simulink library "SUB_ECU_L4_MABX_HW_Interface_PIC_PB"  (R2018a)
settings: Solver=VariableStepAuto  StartTime=0.0  StopTime=10.0  RelTol=1e-3
PostLoadFcn:
  | , if any(exist('dsrtsu_mdlpostloadfcn', 'file') == [2, 3, 6]), try dsrtsu_mdlpostloadfcn('Execute', bdroot); catch fprintf('Error in PostLoadFcn (dsrtsu_mdlpostloadfcn) for model "%s":\n %s\n', bdroot, lasterr); end, end,
undefined symbols (not defined in the file or in its folder): CANR_PROPB_REAX_3_13_CHANNEL_APV, CANR_PROPB_REAX_4_13_CHANNEL_APV, CANR_PROPB_XPR_1_50_CHANNEL_APV, ENUM_CAN_RX_T, ENUM_CAN_TX_T, ENUM_REAX_OPERATION_MODE_T, ENUM_SIGNAL_HEALTH_T, ENUM_XBR_CONTROL_MODE_T, ENUM_XBR_EBI_MODE_T, ENUM_XBR_PASS_THROUGH_ACTIVE_T, ENUM_XBR_PRIORITY_T, ENUM_XPR_INHIBIT_PARK_MANUAL_T, ENUM_XPR_INHIBIT_UNPARK_MANUAL_T, ENUM_XPR_PARK_MANUAL_T, ENUM_XPR_UNPARK_MANUAL_T, PROPB_REAX_1_E4_DES_POS_SIG_SRC_APV, PROPB_REAX_1_E4_DESIRED_OPMODE_APV, PROPB_REAX_1_E4_DESIRED_POSITION_APV, PROPB_REAX_CHANNEL_APV, ptc_matlab_lib
libraries: PTC_MBDS_LIB x293, rtican x158, simulink x61, EmE_MBD_Blockset x38, rti1401lib_dio_type4 x14, simulink_need_slupdate x7, $bdroot x5, rti1401lib_adc_type4 x3, rtmapslib x3, dsa_tcpip_lib x2, SUB_ECU_L4_MABX_HW_Interface_PTC_1571 x1, rtitasklib x1
(part 4 of 49)

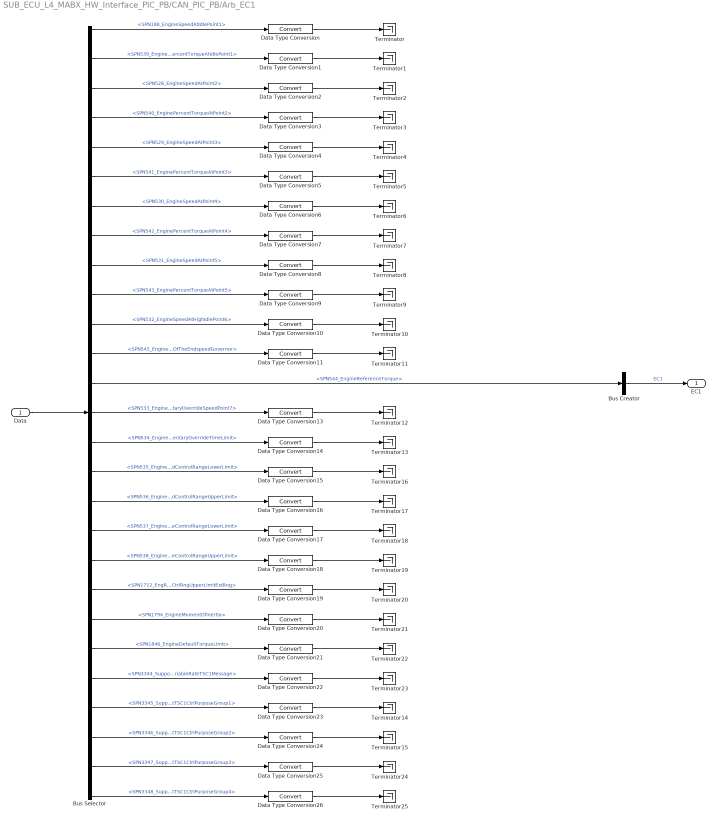
== system SUB_ECU_L4_MABX_HW_Interface_PIC_PB/CAN_PIC_PB/Arb_EC1 ==
  Data : Inport
  Bus Creator : BusCreator  Inputs=1
  Bus Selector : BusSelector  OutputSignals=Signals.SPN188_EngineSpeedAtIdlePoint1,Signals.SPN539_EnginePercentTorqueAtIdlePoint1,Signals.SPN528_EngineSpeedAtPoint2,Signals.SPN540_EnginePercentTorqueAtPoint2,Signals.SPN529_EngineSpeedAtPoint3,Signals.SPN541_EnginePercentTorqueAtPoint3,Signals.SPN530_EngineSpeedAtPoint4,Signals.SPN542_EnginePercentTorqueAtPoint4,Signals.SPN531_EngineSpeedAtPoint5,Signals.SPN543_EnginePercentTorqueAtPoint5,Signals.SPN532_EngineSpeedAtHighIdlePoint6,Signals.SPN545_EngineGainKpOfTheEndspeedGovernor,Signals.SPN544_EngineReferenceTorque,Signals.SPN533_EngineMaximumMomentaryOverrideSpeedPoint7,Signals.SPN534_EngineMaximumMomentaryOverrideTimeLimit,Signals.SPN535_EngineRequestedSpeedControlRangeLowerLimit,Signals.SPN536_EngineRequestedSpeedControlRangeUpperLimit,Signals.SPN537_EngineRequestedTorqueControlRangeLowerLimit,Signals.SPN538_EngineRequestedTorqueControlRangeUpperLimit,Signals.SPN1712_EngRequestedSpeedCtrlRngUpperLimitExtRng,Signals.SPN1794_EngineMomentOfInertia,Signals.SPN1846_EngineDefaultTorqueLimit,Signals.SPN3344_SupportVariableRateTSC1Message,Signals.SPN3345_SupportTSC1CtrlPurposeGroup1,Signals.SPN3346_SupportTSC1CtrlPurposeGroup2,Signals.SPN3347_SupportTSC1CtrlPurposeGroup3,Signals.SPN3348_SupportTSC1CtrlPurposeGroup4
  Data Type Conversion{,1..11,13..26} (26 alike) : DataTypeConversion  SaturateOnIntegerOverflow=on
  Terminator{,1..25} (26 alike) : Terminator
      settings: InitFcn=|
      | try
      |    MBDS_BlockCallback('Update', gcb);
      | end
  EC1 : Outport
  wires:
  Data/1 -> Bus Selector/1
  Bus Selector/1 -> Data Type Conversion/1  "<SPN188_EngineSpeedAtIdlePoint1>"
  Bus Selector/12 -> Data Type Conversion11/1  "<SPN545_EngineGainKpOfTheEndspeedGovernor>"
  Bus Selector/2 -> Data Type Conversion1/1  "<SPN539_EnginePercentTorqueAtIdlePoint1>"
  Bus Selector/3 -> Data Type Conversion2/1  "<SPN528_EngineSpeedAtPoint2>"
  Bus Selector/4 -> Data Type Conversion3/1  "<SPN540_EnginePercentTorqueAtPoint2>"
  Bus Selector/5 -> Data Type Conversion4/1  "<SPN529_EngineSpeedAtPoint3>"
  Bus Selector/6 -> Data Type Conversion5/1  "<SPN541_EnginePercentTorqueAtPoint3>"
  Bus Selector/7 -> Data Type Conversion6/1  "<SPN530_EngineSpeedAtPoint4>"
  Bus Selector/8 -> Data Type Conversion7/1  "<SPN542_EnginePercentTorqueAtPoint4>"
  Bus Selector/9 -> Data Type Conversion8/1  "<SPN531_EngineSpeedAtPoint5>"
  Bus Selector/10 -> Data Type Conversion9/1  "<SPN543_EnginePercentTorqueAtPoint5>"
  Bus Selector/11 -> Data Type Conversion10/1  "<SPN532_EngineSpeedAtHighIdlePoint6>"
  Bus Selector/13 -> Bus Creator/1  "<SPN544_EngineReferenceTorque>"
  Bus Selector/14 -> Data Type Conversion13/1  "<SPN533_EngineMaximumMomentaryOverrideSpeedPoint7>"
  Bus Selector/15 -> Data Type Conversion14/1  "<SPN534_EngineMaximumMomentaryOverrideTimeLimit>"
  Bus Selector/16 -> Data Type Conversion15/1  "<SPN535_EngineRequestedSpeedControlRangeLowerLimit>"
  Bus Selector/17 -> Data Type Conversion16/1  "<SPN536_EngineRequestedSpeedControlRangeUpperLimit>"
  Bus Selector/18 -> Data Type Conversion17/1  "<SPN537_EngineRequestedTorqueControlRangeLowerLimit>"
  Bus Selector/19 -> Data Type Conversion18/1  "<SPN538_EngineRequestedTorqueControlRangeUpperLimit>"
  Bus Selector/20 -> Data Type Conversion19/1  "<SPN1712_EngRequestedSpeedCtrlRngUpperLimitExtRng>"
  Bus Selector/21 -> Data Type Conversion20/1  "<SPN1794_EngineMomentOfInertia>"
  Bus Selector/22 -> Data Type Conversion21/1  "<SPN1846_EngineDefaultTorqueLimit>"
  Bus Selector/23 -> Data Type Conversion22/1  "<SPN3344_SupportVariableRateTSC1Message>"
  Bus Selector/24 -> Data Type Conversion23/1  "<SPN3345_SupportTSC1CtrlPurposeGroup1>"
  Bus Selector/25 -> Data Type Conversion24/1  "<SPN3346_SupportTSC1CtrlPurposeGroup2>"
  Bus Selector/26 -> Data Type Conversion25/1  "<SPN3347_SupportTSC1CtrlPurposeGroup3>"
  Bus Selector/27 -> Data Type Conversion26/1  "<SPN3348_SupportTSC1CtrlPurposeGroup4>"
  Data Type Conversion/1 -> Terminator/1
  Data Type Conversion1/1 -> Terminator1/1
  Data Type Conversion2/1 -> Terminator2/1
  Data Type Conversion3/1 -> Terminator3/1
  Data Type Conversion6/1 -> Terminator6/1
  Data Type Conversion5/1 -> Terminator5/1
  Data Type Conversion7/1 -> Terminator7/1
  Data Type Conversion4/1 -> Terminator4/1
  Data Type Conversion9/1 -> Terminator9/1
  Data Type Conversion10/1 -> Terminator10/1
  Data Type Conversion13/1 -> Terminator12/1
  Data Type Conversion14/1 -> Terminator13/1
  Data Type Conversion15/1 -> Terminator16/1
  Data Type Conversion8/1 -> Terminator8/1
  Data Type Conversion11/1 -> Terminator11/1
  Data Type Conversion20/1 -> Terminator21/1
  Data Type Conversion22/1 -> Terminator23/1
  Data Type Conversion23/1 -> Terminator14/1
  Data Type Conversion17/1 -> Terminator18/1
  Data Type Conversion16/1 -> Terminator17/1
  Data Type Conversion21/1 -> Terminator22/1
  Data Type Conversion18/1 -> Terminator19/1
  Data Type Conversion19/1 -> Terminator20/1
  Data Type Conversion26/1 -> Terminator25/1
  Data Type Conversion25/1 -> Terminator24/1
  Data Type Conversion24/1 -> Terminator15/1
  Bus Creator/1 -> EC1/1  "EC1"

== system SUB_ECU_L4_MABX_HW_Interface_PIC_PB/CAN_PIC_PB/Arb_PropB_REAX_3 ==
  Data : Inport
  Bus Selector : BusSelector  OutputSignals=Signals.PropB_REAX_3_CurrentOperatingMode,Signals.PropB_REAX_3_ReqOperatingMode,Signals.PropB_REAX_3_StatusErrMsg,Signals.PropB_REAX_3_HandwheelTorque,Signals.PropB_REAX_3_HandwheelVelocity,Signals.PropB_REAX_3_PullCompensation
  Data Type Conversion{,1..5} (6 alike) : DataTypeConversion  SaturateOnIntegerOverflow=on
  Terminator{,1..5} (6 alike) : Terminator
      settings: InitFcn=|
      | try
      |    MBDS_BlockCallback('Update', gcb);
      | end
  wires:
  Data/1 -> Bus Selector/1
  Bus Selector/2 -> Data Type Conversion1/1  "<PropB_REAX_3_ReqOperatingMode>"
  Bus Selector/4 -> Data Type Conversion3/1  "<PropB_REAX_3_HandwheelTorque>"
  Bus Selector/3 -> Data Type Conversion2/1  "<PropB_REAX_3_StatusErrMsg>"
  Bus Selector/1 -> Data Type Conversion/1  "<PropB_REAX_3_CurrentOperatingMode>"
  Bus Selector/5 -> Data Type Conversion4/1  "<PropB_REAX_3_HandwheelVelocity>"
  Bus Selector/6 -> Data Type Conversion5/1  "<PropB_REAX_3_PullCompensation>"
  Data Type Conversion/1 -> Terminator/1
  Data Type Conversion1/1 -> Terminator1/1
  Data Type Conversion2/1 -> Terminator2/1
  Data Type Conversion3/1 -> Terminator3/1
  Data Type Conversion4/1 -> Terminator4/1
  Data Type Conversion5/1 -> Terminator5/1

== system SUB_ECU_L4_MABX_HW_Interface_PIC_PB/CAN_PIC_PB/Arb_PropB_REAX_4 ==
  Data : Inport
  Bus Selector : BusSelector  OutputSignals=Signals.PropB_REAX_4_AbsSteeringPosValid,Signals.PropB_REAX_4_PositionIndexValid,Signals.PropB_REAX_4_DriverControlledEffortsEnabled,Signals.PropB_REAX_4_ControlOperatingMode,Signals.PropB_REAX_4_SystemMode,Signals.PropB_REAX_4_PercHandwheelTorque,Signals.PropB_REAX_4_AbsSteeringAngle,Signals.PropB_REAX_4_PercMotorTorque
  Data Type Conversion{,1..7} (8 alike) : DataTypeConversion  SaturateOnIntegerOverflow=on
  Terminator{,1..7} (8 alike) : Terminator
      settings: InitFcn=|
      | try
      |    MBDS_BlockCallback('Update', gcb);
      | end
  wires:
  Data/1 -> Bus Selector/1
  Bus Selector/4 -> Data Type Conversion3/1  "<PropB_REAX_4_ControlOperatingMode>"
  Bus Selector/3 -> Data Type Conversion2/1  "<PropB_REAX_4_DriverControlledEffortsEnabled>"
  Bus Selector/5 -> Data Type Conversion4/1  "<PropB_REAX_4_SystemMode>"
  Bus Selector/2 -> Data Type Conversion/1  "<PropB_REAX_4_PositionIndexValid>"
  Bus Selector/1 -> Data Type Conversion1/1  "<PropB_REAX_4_AbsSteeringPosValid>"
  Bus Selector/6 -> Data Type Conversion5/1  "<PropB_REAX_4_PercHandwheelTorque>"
  Bus Selector/7 -> Data Type Conversion6/1  "<PropB_REAX_4_AbsSteeringAngle>"
  Bus Selector/8 -> Data Type Conversion7/1  "<PropB_REAX_4_PercMotorTorque>"
  Data Type Conversion1/1 -> Terminator/1
  Data Type Conversion/1 -> Terminator1/1
  Data Type Conversion2/1 -> Terminator2/1
  Data Type Conversion3/1 -> Terminator3/1
  Data Type Conversion4/1 -> Terminator4/1
  Data Type Conversion5/1 -> Terminator5/1
  Data Type Conversion6/1 -> Terminator6/1
  Data Type Conversion7/1 -> Terminator7/1

== system SUB_ECU_L4_MABX_HW_Interface_PIC_PB/CAN_PIC_PB/CAN1_RX_TPCM_FF_00 ==
  Constant : Constant  Value=ENUM_CAN_RX_T.RX_CAN_1
  Multiport_Switch : MultiPortSwitch  DataPortOrder=Specify indices  DataPortIndices={ENUM_CAN_RX_T.RX_CAN_1, ENUM_CAN_RX_T.RX_CAN_2, ENUM_CAN_RX_T.RX_CAN_3, ENUM_CAN_RX_T.RX_CAN_4, ENUM_CAN_RX_T.RX_CAN_5, ENUM_CAN_RX_T.RX_CAN_6}  DataPortForDefault=Additional data port  SaturateOnIntegerOverflow=on  InputSameDT=on
      settings: AttributesFormatString=Zero-based indexing: %<zeroidx>
  RX_CAN_1 : Subsystem
  SelectChannel : Subsystem
  Terminator{,1..4} (5 alike) : Terminator
      settings: InitFcn=|
      | try
      |    MBDS_BlockCallback('Update', gcb);
      | end
  TPCM_FF_00 : Outport
  wires:
  Multiport_Switch/1 -> TPCM_FF_00/1
  SelectChannel/2(CAN2) -> Terminator/1
  SelectChannel/3(CAN3) -> Terminator1/1
  SelectChannel/4(CAN4) -> Terminator2/1
  SelectChannel/5(CAN5) -> Terminator3/1
  SelectChannel/6(CAN6) -> Terminator4/1
  RX_CAN_1/1(TPCM_FF_00) -> Multiport_Switch/2, Multiport_Switch/3, Multiport_Switch/4, Multiport_Switch/5, Multiport_Switch/6, Multiport_Switch/7, Multiport_Switch/8
  SelectChannel/1(CAN1) -> RX_CAN_1/1(Enable)
  Constant/1 -> Multiport_Switch/1, SelectChannel/1(In1)

== system SUB_ECU_L4_MABX_HW_Interface_PIC_PB/CAN_PIC_PB/CAN1_RX_TPDT_FF_00 ==
  Constant : Constant  Value=ENUM_CAN_RX_T.RX_CAN_1
  Multiport_Switch : MultiPortSwitch  DataPortOrder=Specify indices  DataPortIndices={ENUM_CAN_RX_T.RX_CAN_1, ENUM_CAN_RX_T.RX_CAN_2, ENUM_CAN_RX_T.RX_CAN_3, ENUM_CAN_RX_T.RX_CAN_4, ENUM_CAN_RX_T.RX_CAN_5, ENUM_CAN_RX_T.RX_CAN_6}  DataPortForDefault=Additional data port  SaturateOnIntegerOverflow=on  InputSameDT=on
      settings: AttributesFormatString=Zero-based indexing: %<zeroidx>
  RX_CAN_1 : Subsystem
  SelectChannel : Subsystem
  Terminator{,1..4} (5 alike) : Terminator
      settings: InitFcn=|
      | try
      |    MBDS_BlockCallback('Update', gcb);
      | end
  TPDT_FF_00 : Outport
  wires:
  Constant/1 -> SelectChannel/1(In1), Multiport_Switch/1
  SelectChannel/1(CAN1) -> RX_CAN_1/1(Enable)
  RX_CAN_1/1(TPDT_FF_00) -> Multiport_Switch/8, Multiport_Switch/7, Multiport_Switch/6, Multiport_Switch/5, Multiport_Switch/4, Multiport_Switch/3, Multiport_Switch/2
  SelectChannel/6(CAN6) -> Terminator4/1
  SelectChannel/5(CAN5) -> Terminator3/1
  SelectChannel/4(CAN4) -> Terminator2/1
  SelectChannel/3(CAN3) -> Terminator1/1
  SelectChannel/2(CAN2) -> Terminator/1
  Multiport_Switch/1 -> TPDT_FF_00/1

== system SUB_ECU_L4_MABX_HW_Interface_PIC_PB/CAN_PIC_PB/CAN_RX_ACC1_2A ==
  Constant : Constant  Value=boolean(1)
  RX_CAN_1 : Subsystem
  ACC1_2A : Outport
  wires:
  Constant/1 -> RX_CAN_1/1(Enable)
  RX_CAN_1/1(ACC1_2A) -> ACC1_2A/1

== system SUB_ECU_L4_MABX_HW_Interface_PIC_PB/CAN_PIC_PB/CAN_RX_AEBS1_2A ==
  Constant : Constant  Value=boolean(1)
  RX_CAN_1 : Subsystem
  AEBS1_2A : Outport
  wires:
  RX_CAN_1/1(AEBS1_2A) -> AEBS1_2A/1
  Constant/1 -> RX_CAN_1/1(Enable)

== system SUB_ECU_L4_MABX_HW_Interface_PIC_PB/CAN_PIC_PB/CAN_RX_AIR1_31 ==
  Constant : Constant  Value=boolean(1)
  RX_CAN_1 : Subsystem
  AIR1_31 : Outport
  wires:
  Constant/1 -> RX_CAN_1/1(Enable)
  RX_CAN_1/1(AIR1_31) -> AIR1_31/1

== system SUB_ECU_L4_MABX_HW_Interface_PIC_PB/CAN_PIC_PB/CAN_RX_AMB_00 ==
  Constant : Constant  Value=boolean(1)
  RX_CAN_1 : Subsystem
  AMB_00 : Outport
  wires:
  RX_CAN_1/1(AMB_00) -> AMB_00/1
  Constant/1 -> RX_CAN_1/1(Enable)

== system SUB_ECU_L4_MABX_HW_Interface_PIC_PB/CAN_PIC_PB/CAN_RX_B2_31 ==
  Constant : Constant
  RX_CAN_4 : Subsystem
  B2_00 : Outport
  wires:
  Constant/1 -> RX_CAN_4/1(Enable)
  RX_CAN_4/1(B2_31) -> B2_00/1

== system SUB_ECU_L4_MABX_HW_Interface_PIC_PB/CAN_PIC_PB/CAN_RX_Bendix_RADAR_Tracks ==
  Constant : Constant  Value=boolean(0)
  RX_CAN_1 : Subsystem
  Bendix_RADAR_Tracks : Outport
  wires:
  Constant/1 -> RX_CAN_1/1(Enable)
  RX_CAN_1/1(Bendix_RADAR_Tracks) -> Bendix_RADAR_Tracks/1

== system SUB_ECU_L4_MABX_HW_Interface_PIC_PB/CAN_PIC_PB/CAN_RX_CCVS1_00 ==
  Constant : Constant  Value=boolean(1)
  RX_CAN_1 : Subsystem
  CCVS1_0 : Outport
  wires:
  RX_CAN_1/1(CCVS1_0) -> CCVS1_0/1
  Constant/1 -> RX_CAN_1/1(Enable)

== system SUB_ECU_L4_MABX_HW_Interface_PIC_PB/CAN_PIC_PB/CAN_RX_CCVS1_31 ==
  Constant : Constant  Value=boolean(1)
  RX_CAN_1 : Subsystem
  CCVS1_31 : Outport
  wires:
  RX_CAN_1/1(CCVS1_31_) -> CCVS1_31/1
  Constant/1 -> RX_CAN_1/1(Enable)

== system SUB_ECU_L4_MABX_HW_Interface_PIC_PB/CAN_PIC_PB/CAN_RX_COGSOGRapidUpdate_01 ==
  Constant : Constant
  RX_CAN_4 : Subsystem
  COGSOGRapidUpdate_01 : Outport
  wires:
  RX_CAN_4/1(COGSOGRapidUpdate_01) -> COGSOGRapidUpdate_01/1
  Constant/1 -> RX_CAN_4/1(Enable)

== system SUB_ECU_L4_MABX_HW_Interface_PIC_PB/CAN_PIC_PB/CAN_RX_CVW_0B ==
  Constant : Constant  Value=boolean(1)
  RX_CAN_1 : Subsystem
  CVW_0B : Outport
  wires:
  RX_CAN_1/1(CVW_0B) -> CVW_0B/1
  Constant/1 -> RX_CAN_1/1(Enable)

== system SUB_ECU_L4_MABX_HW_Interface_PIC_PB/CAN_PIC_PB/CAN_RX_EBC1_0B ==
  Constant1 : Constant  Value=boolean(1)
  RX_CAN_1_EBC1 : Subsystem
  EBC1_0B : Outport
  wires:
  RX_CAN_1_EBC1/1(EBC1_0B_) -> EBC1_0B/1
  Constant1/1 -> RX_CAN_1_EBC1/1(Enable)

== system SUB_ECU_L4_MABX_HW_Interface_PIC_PB/CAN_PIC_PB/CAN_RX_EBC1_8B ==
  Constant1 : Constant  Value=boolean(1)
  RX_CAN_5_EBC1 : Subsystem
  EBC1_8B : Outport
  wires:
  Constant1/1 -> RX_CAN_5_EBC1/1(Enable)
  RX_CAN_5_EBC1/1(EBC1_8B) -> EBC1_8B/1

== system SUB_ECU_L4_MABX_HW_Interface_PIC_PB/CAN_PIC_PB/CAN_RX_EBC2_0B ==
  Enable_RX_EBC2_0B : Constant  Value=boolean(1)
  RX_CAN_1 : Subsystem
  EBC2_0B : Outport
  wires:
  RX_CAN_1/1(EBC2_0B) -> EBC2_0B/1
  Enable_RX_EBC2_0B/1 -> RX_CAN_1/1(Enable)

== system SUB_ECU_L4_MABX_HW_Interface_PIC_PB/CAN_PIC_PB/CAN_RX_EC1_00 ==
  TPCM_BAM_CAN1 : Inport
  TPDT_BAM_CAN1 : Inport  Port=2
  timeStamp : Inport  Port=3
  Bus Creator : BusCreator  Inputs=5
  Bus Selector13 : BusSelector  OutputSignals=RX_status
  Bus Selector5 : BusSelector  OutputSignals=Signals.TPCM_BAM.SPN2569_ParameterGroupNumber
  CAN_RX_EC1_00 : Subsystem  TreatAsAtomicUnit=on
  Constant2 : Constant  Value=uint32(hex2dec('FEE3'))
  Decode_EC1 : PTC_MBDS_LIB/J1939/Decoders/Decode_EC1  PTC_MBDS_BlockVersion=5.41  PTC_BlockType=PTC_MBDS_Decode_EC1
      settings: SourceProductName=PACCAR Technical Center MBDS Library
  EQ1 : PTC_MBDS_LIB/MBDS Standard Library/Basic Operations/Logic and Bit Operations/EQ  InputSameDT=on  PTC_MBDS_BlockVersion=5.41  PTC_BlockType=PTC_MBDS_EQ
      settings: SourceProductName=PACCAR Technical Center MBDS Library
  Logical Operator : Logic  AllPortsSameDT=off  OutDataTypeStr=boolean
  EC1_00 : Outport
  wires:
  Bus Selector13/1 -> Logical Operator/1  "<RX_status>"
  [TPDT_BAM_CAN1] -> Bus Selector13/1
  Bus Selector5/1 -> EQ1/1  "<SPN2569_ParameterGroupNumber>"
  [TPCM_BAM_CAN1] -> Bus Selector5/1
  EQ1/1 -> Logical Operator/2
  Constant2/1 -> EQ1/2
  TPCM_BAM_CAN1/1 -> [TPCM_BAM_CAN1]
  [TPCM_BAM_CAN1] -> CAN_RX_EC1_00/1(TPCM)
  [TPDT_BAM_CAN1] -> CAN_RX_EC1_00/2(TPDT)
  [RX_time] -> Bus Creator/4
  [Signals] -> Bus Creator/1
  [RX_status] -> Bus Creator/3
  [RawData] -> Bus Creator/2
  [RX_delta_time] -> Bus Creator/5
  TPDT_BAM_CAN1/1 -> [TPDT_BAM_CAN1]
  Bus Creator/1 -> EC1_00/1
  CAN_RX_EC1_00/1(RawData) -> [RawData], Decode_EC1/1
  CAN_RX_EC1_00/3(RX_time) -> [RX_time]
  CAN_RX_EC1_00/4(RX_delta_time) -> [RX_delta_time]
  CAN_RX_EC1_00/2(RX_status) -> [RX_status]
  Decode_EC1/1 -> [Signals]
  Logical Operator/1 -> CAN_RX_EC1_00/Enable
  timeStamp/1 -> CAN_RX_EC1_00/3(timeStamp)

== system SUB_ECU_L4_MABX_HW_Interface_PIC_PB/CAN_PIC_PB/CAN_RX_EEC1_00 ==
  Enable_RX_EEC1_00 : Constant  Value=boolean(1)
  RX_CAN_1 : Subsystem
  EEC1_00 : Outport
  wires:
  RX_CAN_1/1(EEC1_00) -> EEC1_00/1
  Enable_RX_EEC1_00/1 -> RX_CAN_1/1(Enable)

== system SUB_ECU_L4_MABX_HW_Interface_PIC_PB/CAN_PIC_PB/CAN_RX_EEC2_00 ==
  Enable_RX_EEC2_00 : Constant  Value=boolean(1)
  RX_CAN_2 : Subsystem
  EEC2_00 : Outport
  wires:
  Enable_RX_EEC2_00/1 -> RX_CAN_2/1(Enable)
  RX_CAN_2/1(EEC2_00) -> EEC2_00/1

== system SUB_ECU_L4_MABX_HW_Interface_PIC_PB/CAN_PIC_PB/CAN_RX_EEC3_00 ==
  Enable_RX_EEC3_00 : Constant  Value=boolean(1)
  RX_CAN_1 : Subsystem
  EEC3_00 : Outport
  wires:
  RX_CAN_1/1(EEC3_00) -> EEC3_00/1
  Enable_RX_EEC3_00/1 -> RX_CAN_1/1(Enable)

== system SUB_ECU_L4_MABX_HW_Interface_PIC_PB/CAN_PIC_PB/CAN_RX_ETC2_03 ==
  Enable_RX_ETC2_03 : Constant  Value=boolean(1)
  RX_CAN_1 : Subsystem
  ETC2_03 : Outport
  wires:
  RX_CAN_1/1(ETC2_03) -> ETC2_03/1
  Enable_RX_ETC2_03/1 -> RX_CAN_1/1(Enable)

== system SUB_ECU_L4_MABX_HW_Interface_PIC_PB/CAN_PIC_PB/CAN_RX_GNSSDOPs_00 ==
  Constant : Constant  Value=0
  RX_CAN_4 : Subsystem
  GNSSDOPs_00 : Outport
  wires:
  RX_CAN_4/1(GNSSDOPs_00) -> GNSSDOPs_00/1
  Constant/1 -> RX_CAN_4/1(Enable)

== system SUB_ECU_L4_MABX_HW_Interface_PIC_PB/CAN_PIC_PB/CAN_RX_HRW_0B ==
  Enable_HRW_RX_0B : Constant  Value=boolean(1)
  RX_CAN_1 : Subsystem
  HRW_0B : Outport
  wires:
  Enable_HRW_RX_0B/1 -> RX_CAN_1/1(Enable)
  RX_CAN_1/1(HRW_0B_) -> HRW_0B/1

== system SUB_ECU_L4_MABX_HW_Interface_PIC_PB/CAN_PIC_PB/CAN_RX_PROPB_REAX_2_13 ==
  In1 : Inport
  Bus Selector : BusSelector  OutputSignals=EnablePropB_ReAX_CAN2,EnablePropB_ReAX_CAN6
  RX_CAN_2 : Subsystem
  RX_CAN_6 : Subsystem
  Switch : Switch  Criteria=u2 ~= 0
  PROPB_REAX_2_13 : Outport
  wires:
  RX_CAN_2/1(PROPB_REAX_2_13) -> Switch/1
  In1/1 -> Bus Selector/1
  Bus Selector/1 -> Switch/2, RX_CAN_2/1(Enable)  "<EnablePropB_ReAX_CAN2>"
  RX_CAN_6/1(PROPB_REAX_2_13) -> Switch/3
  Switch/1 -> PROPB_REAX_2_13/1
  Bus Selector/2 -> RX_CAN_6/1(Enable)  "<EnablePropB_ReAX_CAN6>"

== system SUB_ECU_L4_MABX_HW_Interface_PIC_PB/CAN_PIC_PB/CAN_RX_PROPB_REAX_3_13 ==
  Constant : Constant  Value=CANR_PROPB_REAX_3_13_CHANNEL_APV
  Multiport_Switch : MultiPortSwitch  DataPortOrder=Specify indices  DataPortIndices={ENUM_CAN_RX_T.RX_CAN_1, ENUM_CAN_RX_T.RX_CAN_2, ENUM_CAN_RX_T.RX_CAN_3, ENUM_CAN_RX_T.RX_CAN_4, ENUM_CAN_RX_T.RX_CAN_5, ENUM_CAN_RX_T.RX_CAN_6}  DataPortForDefault=Additional data port  SaturateOnIntegerOverflow=on  InputSameDT=on
      settings: AttributesFormatString=Zero-based indexing: %<zeroidx>
  RX_CAN_1 : Subsystem
  RX_CAN_2 : Subsystem
  SelectChannel : Subsystem
  Terminator{1..4} (4 alike) : Terminator
      settings: InitFcn=|
      | try
      |    MBDS_BlockCallback('Update', gcb);
      | end
  PROPB_REAX_3_13 : Outport
  wires:
  Multiport_Switch/1 -> PROPB_REAX_3_13/1
  SelectChannel/2(CAN2) -> RX_CAN_2/1(Enable)
  SelectChannel/3(CAN3) -> Terminator1/1
  SelectChannel/4(CAN4) -> Terminator2/1
  SelectChannel/5(CAN5) -> Terminator3/1
  SelectChannel/6(CAN6) -> Terminator4/1
  SelectChannel/1(CAN1) -> RX_CAN_1/1(Enable)
  Constant/1 -> Multiport_Switch/1, SelectChannel/1(In1)
  RX_CAN_2/1(PROPB_REAX_3_13) -> Multiport_Switch/8, Multiport_Switch/7, Multiport_Switch/6, Multiport_Switch/5, Multiport_Switch/4, Multiport_Switch/3
  RX_CAN_1/1(PROPB_REAX_3_13) -> Multiport_Switch/2

== system SUB_ECU_L4_MABX_HW_Interface_PIC_PB/CAN_PIC_PB/CAN_RX_PROPB_REAX_4_13 ==
  Constant : Constant  Value=CANR_PROPB_REAX_4_13_CHANNEL_APV
  Multiport_Switch : MultiPortSwitch  DataPortOrder=Specify indices  DataPortIndices={ENUM_CAN_RX_T.RX_CAN_1, ENUM_CAN_RX_T.RX_CAN_2, ENUM_CAN_RX_T.RX_CAN_3, ENUM_CAN_RX_T.RX_CAN_4, ENUM_CAN_RX_T.RX_CAN_5, ENUM_CAN_RX_T.RX_CAN_6}  DataPortForDefault=Additional data port  SaturateOnIntegerOverflow=on  InputSameDT=on
      settings: AttributesFormatString=Zero-based indexing: %<zeroidx>
  RX_CAN_1 : Subsystem
  RX_CAN_2 : Subsystem
  SelectChannel : Subsystem
  Terminator{1..4} (4 alike) : Terminator
      settings: InitFcn=|
      | try
      |    MBDS_BlockCallback('Update', gcb);
      | end
  PROPB_REAX_4_13 : Outport
  wires:
  Constant/1 -> SelectChannel/1(In1), Multiport_Switch/1
  SelectChannel/1(CAN1) -> RX_CAN_1/1(Enable)
  SelectChannel/6(CAN6) -> Terminator4/1
  SelectChannel/5(CAN5) -> Terminator3/1
  SelectChannel/4(CAN4) -> Terminator2/1
  SelectChannel/3(CAN3) -> Terminator1/1
  SelectChannel/2(CAN2) -> RX_CAN_2/1(Enable)
  Multiport_Switch/1 -> PROPB_REAX_4_13/1
  RX_CAN_1/1(PROPB_REAX_4_13) -> Multiport_Switch/2
  RX_CAN_2/1(PROPB_REAX_4_13) -> Multiport_Switch/8, Multiport_Switch/7, Multiport_Switch/6, Multiport_Switch/5, Multiport_Switch/4, Multiport_Switch/3

== system SUB_ECU_L4_MABX_HW_Interface_PIC_PB/CAN_PIC_PB/CAN_RX_PROPB_XPR_1_50 ==
  Constant : Constant  Value=CANR_PROPB_XPR_1_50_CHANNEL_APV
  Multiport_Switch : MultiPortSwitch  DataPortOrder=Specify indices  DataPortIndices={ENUM_CAN_RX_T.RX_CAN_1, ENUM_CAN_RX_T.RX_CAN_2, ENUM_CAN_RX_T.RX_CAN_3, ENUM_CAN_RX_T.RX_CAN_4, ENUM_CAN_RX_T.RX_CAN_5, ENUM_CAN_RX_T.RX_CAN_6}  DataPortForDefault=Additional data port  SaturateOnIntegerOverflow=on  InputSameDT=on
      settings: AttributesFormatString=Zero-based indexing: %<zeroidx>
  RX_CAN_1 : Subsystem
  RX_CAN_2 : Subsystem
  SelectChannel : Subsystem
  Terminator{1..4} (4 alike) : Terminator
      settings: InitFcn=|
      | try
      |    MBDS_BlockCallback('Update', gcb);
      | end
  PROPB_XPR_1 : Outport
  wires:
  Constant/1 -> SelectChannel/1(In1), Multiport_Switch/1
  SelectChannel/1(CAN1) -> RX_CAN_1/1(Enable)
  SelectChannel/6(CAN6) -> Terminator4/1
  SelectChannel/5(CAN5) -> Terminator3/1
  SelectChannel/4(CAN4) -> Terminator2/1
  SelectChannel/3(CAN3) -> Terminator1/1
  SelectChannel/2(CAN2) -> RX_CAN_2/1(Enable)
  Multiport_Switch/1 -> PROPB_XPR_1/1
  RX_CAN_2/1(PROPB_XPR_1_50) -> Multiport_Switch/3, Multiport_Switch/4, Multiport_Switch/5, Multiport_Switch/6, Multiport_Switch/7, Multiport_Switch/8
  RX_CAN_1/1(PROPB_XPR_1_50) -> Multiport_Switch/2

== system SUB_ECU_L4_MABX_HW_Interface_PIC_PB/CAN_PIC_PB/CAN_RX_PX2 ==
  Constant : Constant  Value=boolean(0)
  RX_CAN_6 : Subsystem
  PX2_Lane : Outport
  wires:
  Constant/1 -> RX_CAN_6/1(Enable)
  RX_CAN_6/1(PX2_Lane_) -> PX2_Lane/1

== system SUB_ECU_L4_MABX_HW_Interface_PIC_PB/CAN_PIC_PB/CAN_RX_PosRapidUpdate_01 ==
  In1 : Inport
  Constant : Constant  Value=0
  RX_CAN_4 : Subsystem
  PosRapidUpdate_01 : Outport
  wires:
  RX_CAN_4/1(PosRapidUpdate_01) -> PosRapidUpdate_01/1
  Constant/1 -> RX_CAN_4/1(Enable)
  In1/1 -> RX_CAN_4/2(In)

== system SUB_ECU_L4_MABX_HW_Interface_PIC_PB/CAN_PIC_PB/CAN_RX_SSI2_03 ==
  Constant : Constant
  RX_CAN_1 : Subsystem
  SSI2_03 : Outport
  wires:
  RX_CAN_1/1(SSI2_03) -> SSI2_03/1
  Constant/1 -> RX_CAN_1/1(Enable)

== system SUB_ECU_L4_MABX_HW_Interface_PIC_PB/CAN_PIC_PB/CAN_RX_STD_PROPB_PX2_1_E2 ==
  CAN_RX-Enable_PX2_MapLaneEgoLeft : Constant  Value=boolean(0)
  RX_CAN_6 : Subsystem
  PX2_MapLaneEgoLeft : Outport
  wires:
  RX_CAN_6/1(CAN_RX_PX2_MapLaneEgoLeft) -> PX2_MapLaneEgoLeft/1
  CAN_RX-Enable_PX2_MapLaneEgoLeft/1 -> RX_CAN_6/1(Enable)

== system SUB_ECU_L4_MABX_HW_Interface_PIC_PB/CAN_PIC_PB/CAN_RX_STD_PROPB_PX2_1_E3 ==
  CAN_RX-Enable_PX2_MapLaneEgoLeft : Constant  Value=boolean(0)
  RX_CAN_6 : Subsystem
  PX2_MapLaneEgoRight : Outport
  wires:
  CAN_RX-Enable_PX2_MapLaneEgoLeft/1 -> RX_CAN_6/1(Enable)
  RX_CAN_6/1(CAN_RX_PX2_MapLaneEgoRight) -> PX2_MapLaneEgoRight/1

== system SUB_ECU_L4_MABX_HW_Interface_PIC_PB/CAN_PIC_PB/CAN_RX_STD_PROPB_PX2_1_E5 ==
  Constant : Constant  Value=boolean(0)
  RX_CAN_6 : Subsystem
  STD_PROPB_PX2_1_E5 : Outport
  wires:
  RX_CAN_6/1(STD_PROPB_PX2_1_E5) -> STD_PROPB_PX2_1_E5/1
  Constant/1 -> RX_CAN_6/1(Enable)

== system SUB_ECU_L4_MABX_HW_Interface_PIC_PB/CAN_PIC_PB/CAN_RX_SystemTime_01 ==
  Constant : Constant
  RX_CAN_4 : Subsystem
  SystemTime_00 : Outport
  wires:
  RX_CAN_4/1(SystemTime_00) -> SystemTime_00/1
  Constant/1 -> RX_CAN_4/1(Enable)

== system SUB_ECU_L4_MABX_HW_Interface_PIC_PB/CAN_PIC_PB/CAN_RX_TC1_05 ==
  Constant : Constant  Value=boolean(1)
  RX_CAN_5 : Subsystem
  TC1_05 : Outport
  wires:
  Constant/1 -> RX_CAN_5/1(Enable)
  RX_CAN_5/1(TC1_05) -> TC1_05/1

== system SUB_ECU_L4_MABX_HW_Interface_PIC_PB/CAN_PIC_PB/CAN_RX_VDC1_0B ==
  Constant : Constant  Value=boolean(1)
  RX_CAN_1 : Subsystem
  VDC1_0B : Outport
  wires:
  Constant/1 -> RX_CAN_1/1(Enable)
  RX_CAN_1/1(VDC1_0B) -> VDC1_0B/1

== system SUB_ECU_L4_MABX_HW_Interface_PIC_PB/CAN_PIC_PB/CAN_RX_VDC2_0B ==
  Constant : Constant  Value=boolean(1)
  RX_CAN_1 : Subsystem
  VDC2_0B : Outport
  wires:
  Constant/1 -> RX_CAN_1/1(Enable)
  RX_CAN_1/1(VDC2_0B) -> VDC2_0B/1

== system SUB_ECU_L4_MABX_HW_Interface_PIC_PB/CAN_PIC_PB/CAN_RX_VEP1_03 ==
  Constant : Constant
  RX_CAN_1 : Subsystem
  VEP1_03 : Outport
  wires:
  Constant/1 -> RX_CAN_1/1(Enable)
  RX_CAN_1/1(VEP1_03) -> VEP1_03/1

== system SUB_ECU_L4_MABX_HW_Interface_PIC_PB/CAN_PIC_PB/CAN_RX_VI_00 ==
  TPCM_BAM_CAN1 : Inport
  TPDT_BAM_CAN1 : Inport  Port=2
  timeStamp : Inport  Port=3
  Bus Creator : BusCreator  Inputs=5
  Bus Selector13 : BusSelector  OutputSignals=RX_status
  Bus Selector5 : BusSelector  OutputSignals=Signals.TPCM_BAM.SPN2569_ParameterGroupNumber
  CAN_RX_VI_00 : Subsystem  TreatAsAtomicUnit=on
  Constant2 : Constant  Value=uint32(hex2dec('FEEC'))
  Decode_VI : Subsystem
  EQ1 : PTC_MBDS_LIB/MBDS Standard Library/Basic Operations/Logic and Bit Operations/EQ  InputSameDT=on  PTC_MBDS_BlockVersion=5.41  PTC_BlockType=PTC_MBDS_EQ
      settings: SourceProductName=PACCAR Technical Center MBDS Library
  Logical Operator : Logic  AllPortsSameDT=off  OutDataTypeStr=boolean
  VI_00 : Outport
  wires:
  timeStamp/1 -> CAN_RX_VI_00/3(timeStamp)
  Logical Operator/1 -> CAN_RX_VI_00/Enable
  Decode_VI/1(VI) -> [Signals]
  CAN_RX_VI_00/2(RX_status) -> [RX_status]
  CAN_RX_VI_00/4(RX_delta_time) -> [RX_delta_time]
  CAN_RX_VI_00/3(RX_time) -> [RX_time]
  CAN_RX_VI_00/1(RawData) -> Decode_VI/1(RawData), [RawData]
  Bus Creator/1 -> VI_00/1
  TPDT_BAM_CAN1/1 -> [TPDT_BAM_CAN1]
  [RX_delta_time] -> Bus Creator/5
  [RawData] -> Bus Creator/2
  [RX_status] -> Bus Creator/3
  [Signals] -> Bus Creator/1
  [RX_time] -> Bus Creator/4
  [TPDT_BAM_CAN1] -> CAN_RX_VI_00/2(TPDT)
  [TPCM_BAM_CAN1] -> CAN_RX_VI_00/1(TPCM)
  TPCM_BAM_CAN1/1 -> [TPCM_BAM_CAN1]
  Constant2/1 -> EQ1/2
  EQ1/1 -> Logical Operator/2
  [TPCM_BAM_CAN1] -> Bus Selector5/1
  Bus Selector5/1 -> EQ1/1  "<SPN2569_ParameterGroupNumber>"
  [TPDT_BAM_CAN1] -> Bus Selector13/1
  Bus Selector13/1 -> Logical Operator/1  "<RX_status>"

== system SUB_ECU_L4_MABX_HW_Interface_PIC_PB/CAN_PIC_PB/CAN_enable ==
  In1 : Inport
  Bus Creator : BusCreator  Inputs=3
  Bus Selector : BusSelector  OutputSignals=VI_00.Signals.F_Truck1571_VIN_Match,VI_00.Signals.F_Truck166_VIN_Match
  Constant : Constant  Value=PROPB_REAX_CHANNEL_APV
  Constant1 : Constant  Value=ENUM_CAN_RX_T.RX_CAN_2
  Constant2 : Constant  Value=ENUM_CAN_RX_T.RX_CAN_6
  Equal : RelationalOperator  Operator===  OutDataTypeStr=boolean  RndMeth=Simplest
  Equal1 : RelationalOperator  Operator===  OutDataTypeStr=boolean  RndMeth=Simplest
  If_Then_Else : EmE_MBD_Blockset/Signal Routing/If_Then_Else
      settings: SourceProductName=PACCAR EmE MBD Blockset
  Terminator : Terminator
  useGPSSA0 : Constant  Value=boolean(0)
  useGPSSA00 : Constant  Value=boolean(1)
  Out1 : Outport
  wires:
  Bus Creator/1 -> Out1/1
  In1/1 -> Bus Selector/1
  Bus Selector/2 -> Terminator/1  "<F_Truck166_VIN_Match>"
  If_Then_Else/1 -> Bus Creator/3  "useGPS_SA00"
  Bus Selector/1 -> If_Then_Else/1  "<F_Truck1571_VIN_Match>"
  useGPSSA00/1 -> If_Then_Else/2
  useGPSSA0/1 -> If_Then_Else/3
  Equal/1 -> Bus Creator/1  "EnablePropB_ReAX_CAN2"
  Equal1/1 -> Bus Creator/2  "EnablePropB_ReAX_CAN6"
  Constant1/1 -> Equal/1
  Constant/1 -> Equal/2, Equal1/1
  Constant2/1 -> Equal1/2

== system SUB_ECU_L4_MABX_HW_Interface_PIC_PB/CAN_PIC_PB/Decode_PropB_REAX_3 ==
  RawData : Inport  OutDataTypeStr=uint8  PortDimensions=8
  Bus Creator : BusCreator  Inputs=8
  Bus Selector : BusSelector  OutputSignals=byte1
  Bus Selector1 : BusSelector  OutputSignals=byte2
  Bus Selector2 : BusSelector  OutputSignals=byte3,byte4
  Bus Selector3 : BusSelector  OutputSignals=byte5,byte6
  Bus Selector4 : BusSelector  OutputSignals=byte7,byte8
  Demux : Demux  Outputs=8
  MergeBuses : PTC_MBDS_LIB/Extras/Signal Routing/MergeBuses  NumberOfBuses=5  NumberOfBusesPrev=5  PTC_MBDS_BlockVersion=5.41  PTC_BlockType=PTC_MBDS_MergeBuses  DummyParameter=bMKrFwS8rs
      settings: SourceProductName=PACCAR Technical Center MBDS Library
  decode_byte1 : Subsystem
  decode_byte2 : Subsystem
  decode_byte3_byte4 : Subsystem
  decode_byte5_byte6 : Subsystem
  decode_byte7_byte8 : Subsystem
  PROPB_REAX_3 : Outport
  wires:
  RawData/1 -> Demux/1
  Demux/1 -> Bus Creator/1  "byte1"
  Demux/2 -> Bus Creator/2  "byte2"
  Demux/3 -> Bus Creator/3  "byte3"
  Demux/4 -> Bus Creator/4  "byte4"
  Demux/5 -> Bus Creator/5  "byte5"
  Demux/6 -> Bus Creator/6  "byte6"
  Demux/7 -> Bus Creator/7  "byte7"
  Demux/8 -> Bus Creator/8  "byte8"
  Bus Creator/1 -> [RawData]
  MergeBuses/1 -> PROPB_REAX_3/1  "Signals"
  decode_byte2/1(Out) -> MergeBuses/2
  decode_byte1/1(Out) -> MergeBuses/1
  decode_byte3_byte4/1(Out) -> MergeBuses/3
  decode_byte5_byte6/1(Out) -> MergeBuses/4
  decode_byte7_byte8/1(Out) -> MergeBuses/5
  [RawData] -> Bus Selector4/1, Bus Selector3/1, Bus Selector2/1, Bus Selector1/1, Bus Selector/1
  Bus Selector/1 -> decode_byte1/1(byte1)  "<byte1>"
  Bus Selector1/1 -> decode_byte2/1(byte2)  "<byte2>"
  Bus Selector2/1 -> decode_byte3_byte4/1(byte3)  "<byte3>"
  Bus Selector2/2 -> decode_byte3_byte4/2(byte4)  "<byte4>"
  Bus Selector3/1 -> decode_byte5_byte6/1(byte5)  "<byte5>"
  Bus Selector3/2 -> decode_byte5_byte6/2(byte6)  "<byte6>"
  Bus Selector4/1 -> decode_byte7_byte8/1(byte7)  "<byte7>"
  Bus Selector4/2 -> decode_byte7_byte8/2(byte8)  "<byte8>"

== system SUB_ECU_L4_MABX_HW_Interface_PIC_PB/CAN_PIC_PB/Decode_PropB_REAX_4 ==
  RawData : Inport  OutDataTypeStr=uint8  PortDimensions=8
  Bus Creator : BusCreator  Inputs=8
  Bus Selector : BusSelector  OutputSignals=byte1
  Bus Selector1 : BusSelector  OutputSignals=byte2
  Bus Selector2 : BusSelector  OutputSignals=byte3
  Bus Selector3 : BusSelector  OutputSignals=byte5
  Bus Selector4 : BusSelector  OutputSignals=byte6,byte7
  Bus Selector5 : BusSelector  OutputSignals=byte8
  Demux : Demux  Outputs=8
  MergeBuses : PTC_MBDS_LIB/Extras/Signal Routing/MergeBuses  NumberOfBuses=6  NumberOfBusesPrev=6  PTC_MBDS_BlockVersion=5.41  PTC_BlockType=PTC_MBDS_MergeBuses  DummyParameter=d2TEYqDpuU
      settings: SourceProductName=PACCAR Technical Center MBDS Library
  decode_byte1 : Subsystem
  decode_byte2 : Subsystem
  decode_byte3 : Subsystem
  decode_byte5 : Subsystem
  decode_byte6_byte7 : Subsystem
  decode_byte8 : Subsystem
  PROPB_REAX_4 : Outport
  wires:
  [RawData] -> Bus Selector/1, Bus Selector1/1, Bus Selector2/1, Bus Selector3/1, Bus Selector5/1, Bus Selector4/1
  MergeBuses/1 -> PROPB_REAX_4/1  "Signals"
  Bus Creator/1 -> [RawData]
  Demux/8 -> Bus Creator/8  "byte8"
  Demux/7 -> Bus Creator/7  "byte7"
  Demux/6 -> Bus Creator/6  "byte6"
  Demux/5 -> Bus Creator/5  "byte5"
  Demux/4 -> Bus Creator/4  "byte4"
  Demux/3 -> Bus Creator/3  "byte3"
  Demux/2 -> Bus Creator/2  "byte2"
  Demux/1 -> Bus Creator/1  "byte1"
  RawData/1 -> Demux/1
  Bus Selector/1 -> decode_byte1/1(byte1)  "<byte1>"
  Bus Selector1/1 -> decode_byte2/1(byte2)  "<byte2>"
  Bus Selector2/1 -> decode_byte3/1(byte3)  "<byte3>"
  Bus Selector3/1 -> decode_byte5/1(byte5)  "<byte5>"
  Bus Selector4/1 -> decode_byte6_byte7/1(byte6)  "<byte6>"
  Bus Selector4/2 -> decode_byte6_byte7/2(byte7)  "<byte7>"
  Bus Selector5/1 -> decode_byte8/1(byte8)  "<byte8>"
  decode_byte1/1(Out) -> MergeBuses/1
  decode_byte2/1(Out) -> MergeBuses/2
  decode_byte3/1(Out) -> MergeBuses/3
  decode_byte5/1(Out) -> MergeBuses/4
  decode_byte8/1(Out) -> MergeBuses/6
  decode_byte6_byte7/1(Out) -> MergeBuses/5

== system SUB_ECU_L4_MABX_HW_Interface_PIC_PB/DIGITAL/Debounce ==
  In : Inport
  On_Delay_ms : Inport  Port=2
  Off_Delay_ms : Inport  Port=3
  AND : Logic  IconShape=distinctive  AllPortsSameDT=off  OutDataTypeStr=boolean
  AND2 : Logic  IconShape=distinctive  AllPortsSameDT=off  OutDataTypeStr=boolean
  Detect Fall Nonpositive : simulink/Logic and Bit Operations/Detect Fall Nonpositive  vinit=0  OutDataTypeStr=boolean
      settings: SourceProductName=Simulink  SourceProductBaseCode=SL
  Detect Rise Positive : simulink/Logic and Bit Operations/Detect Rise Positive  vinit=0  OutDataTypeStr=boolean
  NOT : Logic  Operator=NOT  IconShape=distinctive  AllPortsSameDT=off  OutDataTypeStr=boolean
  Off Delay : $bdroot/DIGITAL/Debounce/On Delay
  On Delay : Subsystem
  Unit Delay : UnitDelay  SampleTime=-1
  Out : Outport
  wires:
  In/1 -> Detect Rise Positive/1
  AND2/1 -> Out/1
  NOT/1 -> AND/2, AND2/2
  Unit Delay/1 -> Detect Fall Nonpositive/1
  AND/1 -> On Delay/1(In)
  On Delay/1(out) -> Unit Delay/1, AND2/1
  Detect Rise Positive/1 -> AND/1
  Detect Fall Nonpositive/1 -> Off Delay/1
  Off Delay/1 -> NOT/1
  On_Delay_ms/1 -> On Delay/2(time_ms)
  Off_Delay_ms/1 -> Off Delay/2

== system SUB_ECU_L4_MABX_HW_Interface_PIC_PB/DIGITAL/PWM pedal input management ==
  Pedal_1_pwm_freq_raw_value : Inport
  Pedal_1_pwm_dc_raw_value : Inport  Port=2
  Pedal_2_pwm_freq_raw_value : Inport  Port=3
  Pedal_2_pwm_dc_raw_value : Inport  Port=4
  Determine common angle : Subsystem
  Diagnose pedal input signals : Subsystem
  F_PEDAL_TORQUE_SLEW_AT_FAULT : Constant  Value=true
  Fault arbitration : Subsystem
  If_Then_Else : EmE_MBD_Blockset/Signal Routing/If_Then_Else
      settings: SourceProductName=PACCAR EmE MBD Blockset
  Logical Operator6 : Logic  Operator=OR  OutDataTypeStr=boolean
  PEDAL_PWM_SENSOR_DATA_APV.DEFAULT_SLEW_DOWN : Constant  Value=25
  PEDAL_PWM_SENSOR_DATA_APV.DEFAULT_SLEW_UP : Constant  Value=25
  PEDAL_PWM_SENSOR_DATA_APV.DEFAULT_VALUE : Constant  Value=0
  PEDAL_PWM_SENSOR_DATA_APV.DT : Constant  Value=0.01
  PWM signal filtering conversion : Subsystem
  Slew_at_event : EmE_MBD_Blockset/Math Operators/Slew_at_event
      settings: SourceProductName=PACCAR EmE MBD Blockset
  Synchronization check sensor 1 and 2 : Subsystem
  Pedal_pwm_position : Outport
  wires:
  If_Then_Else/1 -> Pedal_pwm_position/1  "Pedal_pwm_position"
  Slew_at_event/2 -> If_Then_Else/2  "Pedal_pwm_angle_common_slewed"
  Slew_at_event/1 -> If_Then_Else/1  "F_Pedal_pwm_fault_slew_enabled"
  F_PEDAL_TORQUE_SLEW_AT_FAULT/1 -> Slew_at_event/Enable
  PEDAL_PWM_SENSOR_DATA_APV.DT/1 -> Slew_at_event/6
  PEDAL_PWM_SENSOR_DATA_APV.DEFAULT_SLEW_DOWN/1 -> Slew_at_event/5
  PEDAL_PWM_SENSOR_DATA_APV.DEFAULT_SLEW_UP/1 -> Slew_at_event/4
  Logical Operator6/1 -> Slew_at_event/1
  Diagnose pedal input signals/1(Pedal_1_pwm_health_state) -> Fault arbitration/1(Pedal_1_pwm_health_state), Determine common angle/1(Pedal_1_pwm_health_state)
  Diagnose pedal input signals/3(Pedal_2_pwm_health_state) -> Fault arbitration/4(Pedal_2_pwm_health_state), Determine common angle/3(Pedal_2_pwm_health_state)
  Diagnose pedal input signals/4(Pedal_synch_data.F_Hard) -> [Pedal_synch_data_F_Hard]
  Diagnose pedal input signals/2(F_Pedal_pwm_sens_total_failure) -> [F_Pedal_pwm_sens_total_failure], Determine common angle/2(F_Pedal_pwm_sens_total_failure)
  [F_Pedal_pwm_sync_fault] -> Diagnose pedal input signals/5(F_Pedal_pwm_sync_fault)
  Pedal_2_pwm_dc_raw_value/1 -> Diagnose pedal input signals/4(Pedal_2_pwm_dc_raw_value)
  Pedal_2_pwm_freq_raw_value/1 -> Diagnose pedal input signals/3(Pedal_2_pwm_freq_raw_value), PWM signal filtering conversion/2(Pedal _2_pwm_dc_raw_value)
  Pedal_1_pwm_dc_raw_value/1 -> Diagnose pedal input signals/2(Pedal_1_pwm_dc_raw_value), PWM signal filtering conversion/1(Pedal _1_pwm_dc_raw_value)
  Pedal_1_pwm_freq_raw_value/1 -> Diagnose pedal input signals/1(Pedal_1_pwm_freq_raw_value)
  Determine common angle/1(Pedal_pwm_angle_common) -> Synchronization check sensor 1 and 2/1(Pedal_pwm_angle_common), Slew_at_event/2, If_Then_Else/3
  [F_Pedal_pwm_sens_total_failure] -> Logical Operator6/1
  [Pedal_synch_data_F_Hard] -> Logical Operator6/2
  Synchronization check sensor 1 and 2/1(F_Pedal_pwm_sync_fault) -> [F_Pedal_pwm_sync_fault]
  Fault arbitration/1(Pedal_1_pwm_angle_arbitrated) -> Determine common angle/4(Pedal_1_pwm_angle_arbitrated)
  Fault arbitration/2(Pedal_2_pwm_angle_arbitrated) -> Determine common angle/5(Pedal_2_pwm_angle_arbitrated)
  PWM signal filtering conversion/2(Pedal_2_pwm_undefault) -> Fault arbitration/5(Pedal_2_pwm_undefault), Synchronization check sensor 1 and 2/3(Pedal_2_pwm_undefault)
  PWM signal filtering conversion/1(Pedal_1_pwm_undefault) -> Fault arbitration/2(Pedal_1_pwm_undefault), Synchronization check sensor 1 and 2/2(Pedal_1_pwm_undefault)
  PEDAL_PWM_SENSOR_DATA_APV.DEFAULT_VALUE/1 -> Slew_at_event/3, Fault arbitration/3(DEFAULT_VALUE), Determine common angle/6(DEFAULT_VALUE)

== system SUB_ECU_L4_MABX_HW_Interface_PIC_PB/DIGITAL/Signal Check ==
  NO : Inport
  NC : Inport  Port=2
  AND : PTC_MBDS_LIB/MBDS Standard Library/Basic Operations/Logic and Bit Operations/AND  BitwiseMode=on  Inputs=1  UseBitMask=on  BitMask=bin2dec('0000000000000001')  OutDataTypeStr=boolean  PTC_MBDS_BlockVersion=5.41  PTC_BlockType=PTC_MBDS_AND
      settings: AttributesFormatString=bitwise  SourceProductName=PACCAR Technical Center MBDS Library
  AND1 : PTC_MBDS_LIB/MBDS Standard Library/Basic Operations/Logic and Bit Operations/AND  BitwiseMode=on  Inputs=1  UseBitMask=on  BitMask=bin2dec('0000000000000001')  OutDataTypeStr=boolean  PTC_MBDS_BlockVersion=5.41  PTC_BlockType=PTC_MBDS_AND
      settings: AttributesFormatString=bitwise  SourceProductName=PACCAR Technical Center MBDS Library
  AND2 : Logic  IconShape=distinctive  AllPortsSameDT=off  OutDataTypeStr=boolean
  Logical Operator : Logic  Operator=NOT  AllPortsSameDT=off  OutDataTypeStr=boolean
  OverrideOperatorEnableSW_Default : Constant  Value=boolean(0)
  RationalityCheck : Subsystem
  Switch : PTC_MBDS_LIB/MBDS Standard Library/Signals & Systems/Signal Routing/Switch  OutDataTypeStr_=Inherit: Inherit via back propagation  SaturateOnIntegerOverflow_=on  InputSameDT_=on  PTC_MBDS_BlockVersion=5.41  PTC_BlockType=PTC_MBDS_Switch
      settings: SourceProductName=PACCAR Technical Center MBDS Library
  Out : Outport
  wires:
  Switch/1 -> Out/1
  Logical Operator/1 -> AND2/1
  AND1/1 -> AND2/2
  NC/1 -> AND1/1
  RationalityCheck/1(DiagPassed) -> Switch/2
  OverrideOperatorEnableSW_Default/1 -> Switch/3
  NO/1 -> AND/1
  AND2/1 -> Switch/1, RationalityCheck/1(UndefaultStatus)
  AND/1 -> Logical Operator/1

== system SUB_ECU_L4_MABX_HW_Interface_PIC_PB/DIGITAL_out/Determine pedal PWM and duty cycle values ==
  APTC_arb_pedal_position : Inport
  AutonomousEnabled : Inport  Port=2
  In : Inport  Port=3
  1-D Lookup Table2 : Lookup_n-D  NumberOfTableDimensions=1  BreakpointsForDimension1=[0 100]  Table=[10 45]  ExtrapMethod=Clip  UseLastTableValue=on  InputSameDT=on
      settings: AttributesFormatString=|
      | X: %<BreakpointsForDimension1>
      | Y: %<Table>
  1-D Lookup Table3 : Lookup_n-D  NumberOfTableDimensions=1  BreakpointsForDimension1=[0 100]  Table=[20 90]  ExtrapMethod=Clip  UseLastTableValue=on  InputSameDT=on
      settings: AttributesFormatString=|
      | X: %<BreakpointsForDimension1>
      | Y: %<Table>
  APTC_PEDAL_A_PWM_FREQ_HZ_APV : Constant  Value=200
  APTC_PEDAL_B_PWM_FREQ_HZ_APV : Constant  Value=200
  Bus Selector4 : BusSelector  OutputSignals=INPUTS.DIO_Bus.Pedal_1_pwm_dc_raw_value
  Bus Selector5 : BusSelector  OutputSignals=INPUTS.DIO_Bus.Pedal_2_pwm_dc_raw_value
  Bus Selector6 : BusSelector  OutputSignals=INPUTS.DIO_Bus.Pedal_1_pwm_freq_raw_value
  Bus Selector7 : BusSelector  OutputSignals=INPUTS.DIO_Bus.Pedal_2_pwm_freq_raw_value
  If_Then_Else{1..2,4..5} (4 alike) : EmE_MBD_Blockset/Signal Routing/If_Then_Else
      settings: SourceProductName=PACCAR EmE MBD Blockset
  Logical Operator : Logic  Operator=NOT  OutDataTypeStr=boolean
  APTC_PWM_pedalA_freq_out : Outport
  APTC_PWM_pedalA_DC_out : Outport  Port=2
  APTC_PWM_pedalB_freq_out : Outport  Port=3
  APTC_PWM_pedalB_DC_out : Outport  Port=4
  wires:
  AutonomousEnabled/1 -> Logical Operator/1
  APTC_PEDAL_A_PWM_FREQ_HZ_APV/1 -> If_Then_Else4/3
  APTC_PEDAL_B_PWM_FREQ_HZ_APV/1 -> If_Then_Else5/3
  Bus Selector6/1 -> If_Then_Else4/2  "<Pedal_1_pwm_freq_raw_value>"
  Bus Selector4/1 -> If_Then_Else1/2  "<Pedal_1_pwm_dc_raw_value>"
  Bus Selector7/1 -> If_Then_Else5/2  "<Pedal_2_pwm_freq_raw_value>"
  Logical Operator/1 -> If_Then_Else5/1, If_Then_Else4/1, If_Then_Else2/1, If_Then_Else1/1
  Bus Selector5/1 -> If_Then_Else2/2  "<Pedal_2_pwm_dc_raw_value>"
  1-D Lookup Table3/1 -> If_Then_Else2/3  "PedalPWMB_DC_out"
  1-D Lookup Table2/1 -> If_Then_Else1/3  "PedalPWMA_DC_out"
  In/1 -> Bus Selector4/1, Bus Selector6/1, Bus Selector7/1, Bus Selector5/1
  APTC_arb_pedal_position/1 -> 1-D Lookup Table2/1, 1-D Lookup Table3/1
  If_Then_Else1/1 -> APTC_PWM_pedalA_DC_out/1
  If_Then_Else2/1 -> APTC_PWM_pedalB_DC_out/1
  If_Then_Else4/1 -> APTC_PWM_pedalA_freq_out/1
  If_Then_Else5/1 -> APTC_PWM_pedalB_freq_out/1

== system SUB_ECU_L4_MABX_HW_Interface_PIC_PB/DIGITAL_out/Shift Control ==
  In : Inport
  Bus Creator1 : BusCreator  Inputs=1
  Bus Selector : BusSelector  OutputSignals=INPUTS.DIO_Bus.ShiftControlDC
  Bus Selector1 : BusSelector  OutputSignals=INPUTS.CAN.ETC2_03.SPN524_TransSelectedGear,INPUTS.CAN.ETC2_03.SPN523_TransCurrentGear
  Compare To Zero : simulink/Logic and Bit Operations/Compare To Zero  relop===  OutDataTypeStr=boolean
  Compare To Zero1 : simulink/Logic and Bit Operations/Compare To Zero  relop===  OutDataTypeStr=boolean
  Constant : Constant  Value=.4
  Constant1 : Constant  Value=0.5
  Constant2 : Constant  Value=false
  F_ALLOW_ETC2_FOR_NEUTRAL_OUTPUT_APV : Constant  Value=true
  If_Then_Else : EmE_MBD_Blockset/Signal Routing/If_Then_Else
      settings: SourceProductName=PACCAR EmE MBD Blockset
  Logical Operator : Logic  OutDataTypeStr=boolean
  Logical Operator1 : Logic  OutDataTypeStr=boolean
  Logical Operator2 : Logic  Operator=OR  OutDataTypeStr=boolean
  Relational Operator : RelationalOperator  OutDataTypeStr=boolean  RndMeth=Nearest
  Relational Operator1 : RelationalOperator  Operator=<=  OutDataTypeStr=boolean  RndMeth=Nearest
  Out : Outport
  wires:
  Constant2/1 -> If_Then_Else/3
  F_ALLOW_ETC2_FOR_NEUTRAL_OUTPUT_APV/1 -> If_Then_Else/1
  If_Then_Else/1 -> Logical Operator2/2
  Logical Operator/1 -> Logical Operator2/1
  Logical Operator1/1 -> If_Then_Else/2
  Compare To Zero1/1 -> Logical Operator1/2
  Compare To Zero/1 -> Logical Operator1/1
  Bus Selector1/2 -> Compare To Zero1/1  "<SPN523_TransCurrentGear>"
  Bus Selector1/1 -> Compare To Zero/1  "<SPN524_TransSelectedGear>"
  Bus Selector/1 -> Relational Operator1/1, Relational Operator/1  "<ShiftControlDC>"
  Bus Creator1/1 -> Out/1
  Logical Operator2/1 -> Bus Creator1/1  "Neutral"
  Constant/1 -> Relational Operator/2
  Relational Operator1/1 -> Logical Operator/2
  Relational Operator/1 -> Logical Operator/1
  In/1 -> Bus Selector/1, Bus Selector1/1
  Constant1/1 -> Relational Operator1/2

== system SUB_ECU_L4_MABX_HW_Interface_PIC_PB/DIGITAL_out/Status Indicator Lights ==
  Outputs : Inport
  AND : Logic  IconShape=distinctive  AllPortsSameDT=off  OutDataTypeStr=boolean
  AND1 : Logic  Inputs=4  AllPortsSameDT=off  OutDataTypeStr=boolean
  AND2 : Logic  IconShape=distinctive  AllPortsSameDT=off  OutDataTypeStr=boolean
  AND3 : Logic  IconShape=distinctive  AllPortsSameDT=off  OutDataTypeStr=boolean
  Bus Selector1 : BusSelector  OutputSignals=INPUTS.PIC_Bus.SupervisorMode,INPUTS.DIO_Bus.EnableSW,10msTask.AutonomousState.AutonomousEnabled,10msTask.AutonomousState.AutonomousOutputEnabled,10msTask.AutonomousState.MABX_Mode
  Constant2 : Constant  Value=2  OutDataTypeStr=uint8
  EQ1 : PTC_MBDS_LIB/MBDS Standard Library/Basic Operations/Logic and Bit Operations/EQ  InputSameDT=on  PTC_MBDS_BlockVersion=5.41  PTC_BlockType=PTC_MBDS_EQ
      settings: SourceProductName=PACCAR Technical Center MBDS Library
  EQ2 : PTC_MBDS_LIB/MBDS Standard Library/Basic Operations/Logic and Bit Operations/EQ  InputSameDT=on  PTC_MBDS_BlockVersion=5.41  PTC_BlockType=PTC_MBDS_EQ
      settings: SourceProductName=PACCAR Technical Center MBDS Library
  Flash : DiscretePulseGenerator  Period=10  PulseWidth=5  SampleTime=0.1
  Manual Ready : Constant  OutDataTypeStr=uint8
  NOT : Logic  Operator=NOT  IconShape=distinctive  AllPortsSameDT=off  OutDataTypeStr=boolean
  NOT1 : Logic  Operator=NOT  IconShape=distinctive  AllPortsSameDT=off  OutDataTypeStr=boolean
  NOT2 : Logic  Operator=NOT  IconShape=distinctive  AllPortsSameDT=off  OutDataTypeStr=boolean
  OR : Logic  Operator=OR  IconShape=distinctive  AllPortsSameDT=off  OutDataTypeStr=boolean
  OR1 : Logic  Operator=OR  IconShape=distinctive  AllPortsSameDT=off  OutDataTypeStr=boolean
  Blue : Outport
  Green : Outport  Port=2
  Red : Outport  Port=3
  wires:
  AND/1 -> OR/1
  Bus Selector1/3 -> AND/1, NOT1/1  "<AutonomousEnabled>"
  Bus Selector1/2 -> AND1/2  "<EnableSW>"
  Manual Ready/1 -> EQ1/1
  Bus Selector1/5 -> EQ2/2  "<MABX_Mode>"
  Bus Selector1/4 -> OR/2  "<AutonomousOutputEnabled>"
  Outputs/1 -> Bus Selector1/1
  Bus Selector1/1 -> EQ1/2  "<SupervisorMode>"
  Constant2/1 -> EQ2/1
  EQ2/1 -> NOT/1, Red/1
  AND2/1 -> Green/1
  NOT/1 -> [NoFault]
  AND1/1 -> Blue/1
  [NoFault] -> AND2/1, AND1/4
  OR/1 -> AND2/2
  NOT1/1 -> AND1/3
  EQ1/1 -> NOT2/1, AND3/2
  [Flash] -> AND/2
  Flash/1 -> AND3/1, [Flash]
  AND3/1 -> OR1/1
  NOT2/1 -> OR1/2
  OR1/1 -> AND1/1
